simulink model "decouplage"  (R2015b)
settings: Solver=VariableStepAuto  StartTime=0.0  StopTime=30  RelTol=1e-3
values from neighbouring files (symbols this model uses):
  K = (Kd^2)/4    (= 2.25)    [commande_robot.m]
  Kd = 3    [commande_robot.m]
  r = R(1)    [commande_robot.m]    (also in sf_loi_avant_RP.m; sf_retour_linearisant_RP.m)
libraries: lib_robotRP x3
settings Model: Creator=chamand  LastModifiedBy=chamand

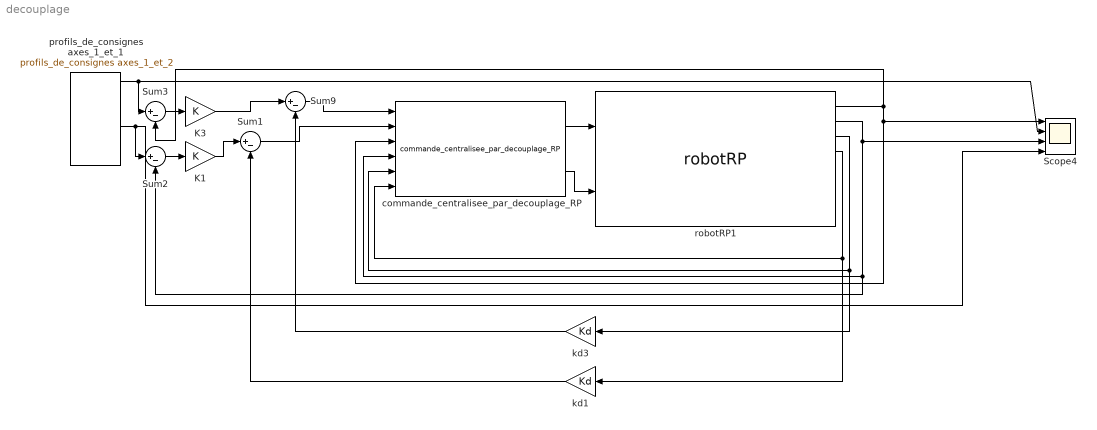
== system decouplage ==
  K1 : Gain  Gain=K
  K3 : Gain  Gain=K
  Scope4 : Scope  NumInputPorts=4
  Sum{1..3,9} (4 alike) : Sum  Inputs=|+-
  commande_centralisee_par_decouplage_RP : lib_robotRP/commande_centralisee_par_decouplage_RP  SystemSampleTime=-1
  kd1 : Gain  Gain=Kd
  kd3 : Gain  Gain=Kd
  profils_de_consignes axes_1_et_1 : lib_robotRP/profils_de_consignes axes_1_et_2
  robotRP1 : lib_robotRP/robotRP  vecteur_theta_dtheta_initial=[0 ; 1/2/r ; 0 ; 0]  m=15  gX=0  gY=-9.81  F1=0  F2=0  H1=0  H2=0  Km_sur_R=0.3  Jm=0.01  Beff=0.0125  r=1/200
  wires:
  robotRP1/2 -> Sum2/2, commande_centralisee_par_decouplage_RP/4, Scope4/3
  profils_de_consignes axes_1_et_1/1 -> Sum3/1, Scope4/2
  robotRP1/3 -> kd3/1, commande_centralisee_par_decouplage_RP/5
  robotRP1/4 -> kd1/1, commande_centralisee_par_decouplage_RP/6
  profils_de_consignes axes_1_et_1/4 -> Sum2/1, Scope4/4
  commande_centralisee_par_decouplage_RP/1 -> robotRP1/1
  commande_centralisee_par_decouplage_RP/2 -> robotRP1/2
  kd3/1 -> Sum9/2
  kd1/1 -> Sum1/2
  K1/1 -> Sum1/1
  Sum1/1 -> commande_centralisee_par_decouplage_RP/2
  K3/1 -> Sum9/1
  Sum9/1 -> commande_centralisee_par_decouplage_RP/1
  Sum2/1 -> K1/1
  Sum3/1 -> K3/1
  robotRP1/1 -> commande_centralisee_par_decouplage_RP/3, Scope4/1, Sum3/2
